simulink model "servomotor"  (Simulink 7.9)
settings: Solver=ode45  StartTime=0.0  StopTime=10.0  RelTol=1e-3
settings Model: Creator=Hetram  LastModifiedBy=Hetram

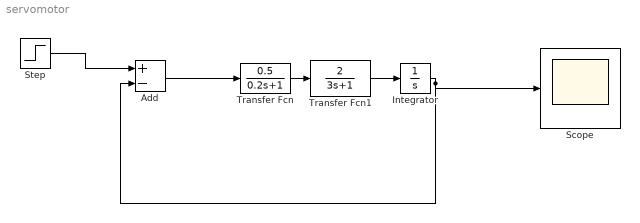
== system servomotor ==
  Add : Sum  Inputs=+-
  Integrator : Integrator
  Scope : Scope
  Step : Step  SampleTime=0
  Transfer Fcn : TransferFcn  Numerator=[0.5]  Denominator=[0.2 1]
  Transfer Fcn1 : TransferFcn  Numerator=[2]  Denominator=[3 1]
  wires:
  Transfer Fcn/1 -> Transfer Fcn1/1
  Transfer Fcn1/1 -> Integrator/1
  Integrator/1 -> Add/2, Scope/1
  Step/1 -> Add/1
  Add/1 -> Transfer Fcn/1
